simulink model "Quadrotor_SMC"  (R2021b)
settings: Solver=VariableStepAuto  StartTime=0.0  StopTime=10  RelTol=1e-3
undefined symbols (not defined in the file): e_Kp, K_rate_d, K_rate_p, Ki, Kp
libraries: simulink x2
settings Model: Creator=Biorobotic_MG  LastModifiedBy=Biorobotic_MG
settings DebuggingCC: UnderSpecifiedDimensionMsg=warning

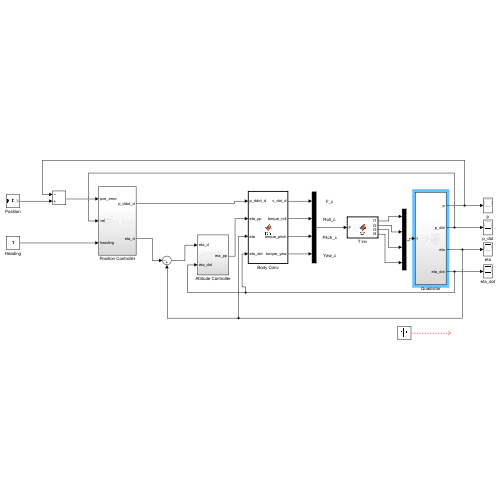
[thumbnail: Simulink's stored preview of the top-level diagram]
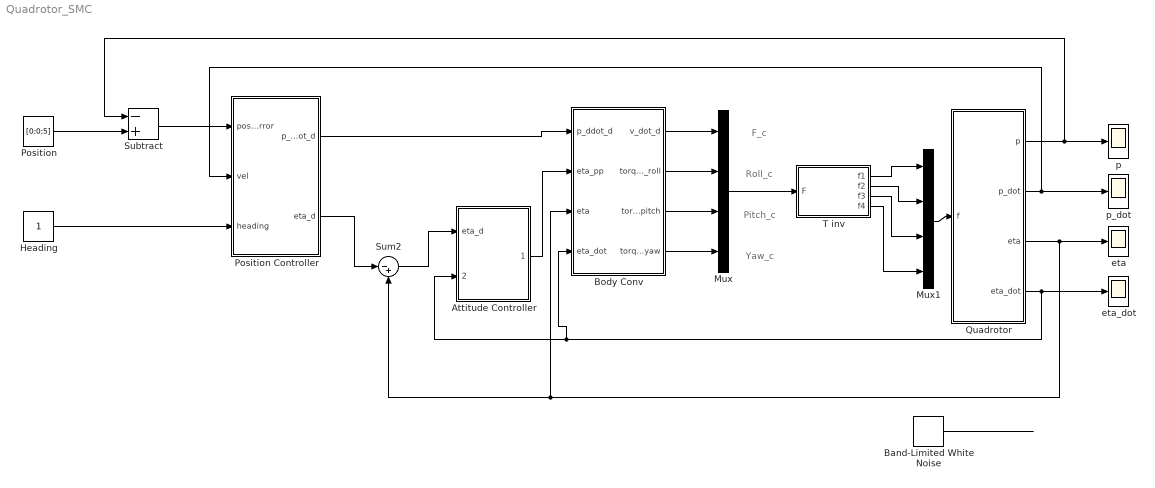
== system Quadrotor_SMC ==
  note: F_c
  note: Roll_c
  note: Pitch_c
  note: Yaw_c
  Attitude Controller : Subsystem
  Band-Limited White Noise : simulink/Sources/Band-Limited White Noise  Cov=[0.01]  Ts=0.1  seed=[23341]
  Body Conv : MATLAB Function  TreatAsAtomicUnit=on
  Heading : Constant
  Mux : Mux
  Mux1 : Mux
  Position : Constant  Value=[0;0;5]  VectorParams1D=off
  Position Controller : Subsystem
  Quadrotor : Subsystem
  Subtract : Sum  Inputs=-+
  Sum2 : Sum  Inputs=|-+
  T inv : MATLAB Function  TreatAsAtomicUnit=on
  eta : Scope
  eta_dot : Scope
  p : Scope
  p_dot : Scope
  wires:
  Quadrotor/1(p) -> Subtract/1, p/1
  Quadrotor/3(eta) -> Sum2/2, Body Conv/3(eta), eta/1
  T inv/1(f1) -> Mux1/1
  T inv/2(f2) -> Mux1/2
  T inv/3(f3) -> Mux1/3
  T inv/4(f4) -> Mux1/4
  Mux1/1 -> Quadrotor/1(f)
  Position/1 -> Subtract/2
  Attitude Controller/1(eta_pp) -> Body Conv/2(eta_pp)
  Subtract/1 -> Position Controller/1(pos_error)
  Heading/1 -> Position Controller/3(heading)
  Position Controller/2(eta_d) -> Sum2/1
  Mux/1 -> T inv/1(F)
  Position Controller/1(p_ddot_d) -> Body Conv/1(p_ddot_d)
  Quadrotor/4(eta_dot) -> eta_dot/1, Body Conv/4(eta_dot), Attitude Controller/2(eta_dot)
  Quadrotor/2(p_dot) -> Position Controller/2(vel), p_dot/1
  Body Conv/4(torque_yaw) -> Mux/4
  Body Conv/3(torque_pitch) -> Mux/3
  Body Conv/2(torque_roll) -> Mux/2
  Body Conv/1(v_dot_d) -> Mux/1
  Sum2/1 -> Attitude Controller/1(eta_d)
  Band-Limited White Noise/1 -> ?

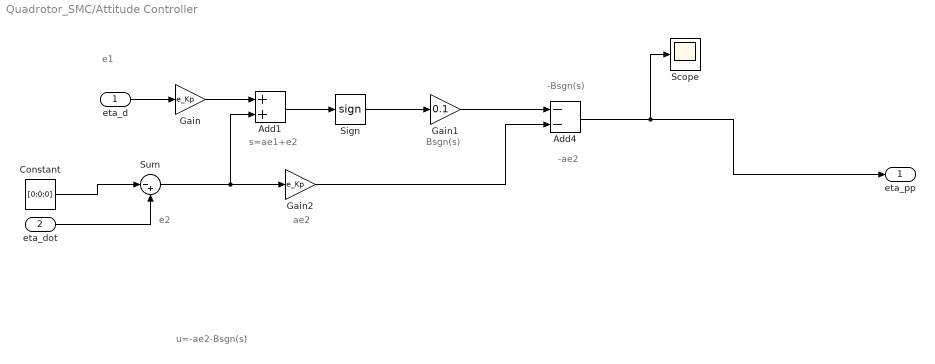
== system Quadrotor_SMC/Attitude Controller ==
  note: -ae2
  note: ae2
  note: e1
  note: e2
  note: s=ae1+e2
  note: Bsgn(s)
  note: -Bsgn(s)
  note: u=-ae2-Bsgn(s)
  eta_d : Inport
  eta_dot : Inport  Port=2
  Add1 : Sum
  Add4 : Sum  Inputs=--
  Constant : Constant  Value=[0;0;0]
  Gain : Gain  Gain=e_Kp
  Gain1 : Gain  Gain=0.1
  Gain2 : Gain  Gain=e_Kp
  Scope : Scope
  Sign : Signum  ZeroCross=off
  Sum : Sum  Inputs=|-+
  eta_pp : Outport
  wires:
  eta_d/1 -> Gain/1
  Gain/1 -> Add1/1
  Sign/1 -> Gain1/1
  Gain1/1 -> Add4/1
  Constant/1 -> Sum/1
  Add4/1 -> Scope/1, eta_pp/1
  Add1/1 -> Sign/1
  eta_dot/1 -> Sum/2
  Sum/1 -> Add1/2, Gain2/1
  Gain2/1 -> Add4/2

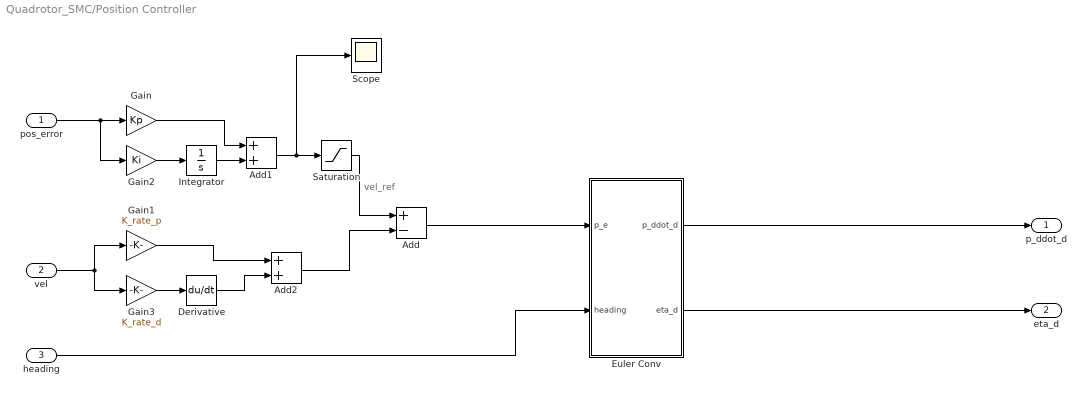
== system Quadrotor_SMC/Position Controller ==
  note: vel_ref
  pos_error : Inport
  vel : Inport  Port=2
  heading : Inport  Port=3
  Add : Sum  Inputs=+-
  Add1 : Sum
  Add2 : Sum
  Derivative : Derivative
  Euler Conv : MATLAB Function  TreatAsAtomicUnit=on
  Gain : Gain  Gain=Kp
  Gain1 : Gain  Gain=K_rate_p
  Gain2 : Gain  Gain=Ki
  Gain3 : Gain  Gain=K_rate_d
  Integrator : Integrator
  Saturation : Saturate  UpperLimit=3  LowerLimit=-3
  Scope : Scope
  p_ddot_d : Outport
  eta_d : Outport  Port=2
  wires:
  pos_error/1 -> Gain2/1, Gain/1
  Euler Conv/1(p_ddot_d) -> p_ddot_d/1
  heading/1 -> Euler Conv/2(heading)
  Gain/1 -> Add1/1
  Gain2/1 -> Integrator/1
  Integrator/1 -> Add1/2
  Gain3/1 -> Derivative/1
  vel/1 -> Gain1/1, Gain3/1
  Gain1/1 -> Add2/1
  Derivative/1 -> Add2/2
  Add2/1 -> Add/2
  Add/1 -> Euler Conv/1(p_e)
  Euler Conv/2(eta_d) -> eta_d/1
  Add1/1 -> Saturation/1, Scope/1
  Saturation/1 -> Add/1

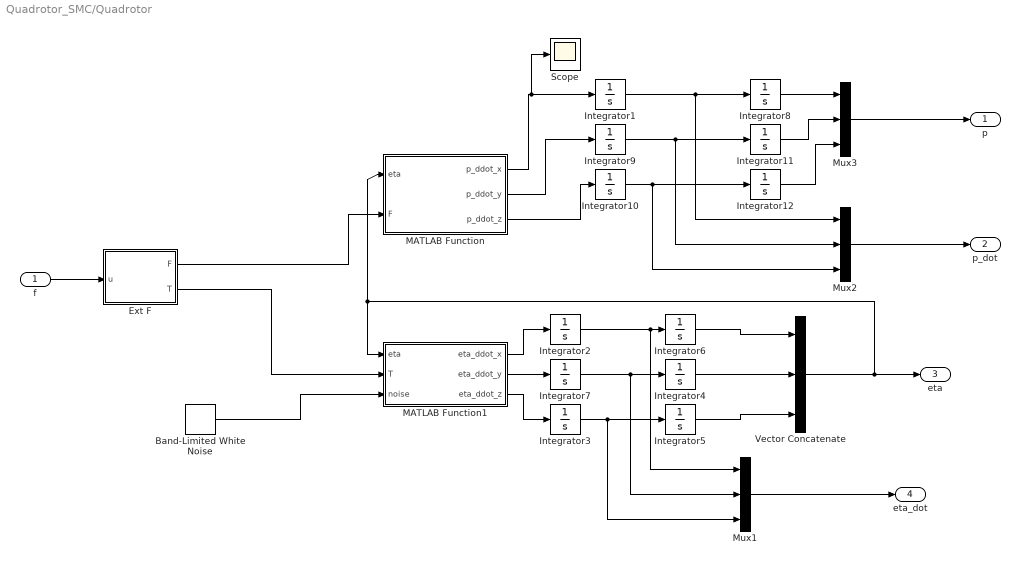
== system Quadrotor_SMC/Quadrotor ==
  f : Inport
  Band-Limited White Noise : simulink/Sources/Band-Limited White Noise  Cov=[0.01]  Ts=0.1  seed=[23341]
  Ext F : MATLAB Function  TreatAsAtomicUnit=on
  Integrator{1..12} (12 alike) : Integrator
  MATLAB Function : MATLAB Function  TreatAsAtomicUnit=on
  MATLAB Function1 : MATLAB Function  TreatAsAtomicUnit=on
  Mux1 : Mux  Inputs=3
  Mux2 : Mux  Inputs=3
  Mux3 : Mux  Inputs=3
  Scope : Scope
  Vector Concatenate : Concatenate  NumInputs=3  Mode=Multidimensional array
  p : Outport
  p_dot : Outport  Port=2
  eta : Outport  Port=3
  eta_dot : Outport  Port=4
  wires:
  Ext F/2(T) -> MATLAB Function1/2(T)
  Ext F/1(F) -> MATLAB Function/2(F)
  f/1 -> Ext F/1(u)
  Integrator10/1 -> Mux2/3, Integrator12/1
  Integrator12/1 -> Mux3/3
  Integrator11/1 -> Mux3/2
  Integrator9/1 -> Mux2/2, Integrator11/1
  Integrator1/1 -> Mux2/1, Integrator8/1
  MATLAB Function/1(p_ddot_x) -> Scope/1, Integrator1/1
  MATLAB Function/2(p_ddot_y) -> Integrator9/1
  MATLAB Function/3(p_ddot_z) -> Integrator10/1
  Integrator8/1 -> Mux3/1
  Mux3/1 -> p/1
  Mux2/1 -> p_dot/1
  Vector Concatenate/1 -> MATLAB Function/1(eta), MATLAB Function1/1(eta), eta/1
  MATLAB Function1/3(eta_ddot_z) -> Integrator3/1
  MATLAB Function1/2(eta_ddot_y) -> Integrator7/1
  Integrator4/1 -> Vector Concatenate/2
  Integrator6/1 -> Vector Concatenate/1
  Integrator2/1 -> Mux1/1, Integrator6/1
  Integrator7/1 -> Mux1/2, Integrator4/1
  Integrator3/1 -> Mux1/3, Integrator5/1
  Integrator5/1 -> Vector Concatenate/3
  MATLAB Function1/1(eta_ddot_x) -> Integrator2/1
  Mux1/1 -> eta_dot/1
  Band-Limited White Noise/1 -> MATLAB Function1/3(noise)

== matlab function Quadrotor_SMC/Quadrotor/MATLAB Function ==
  data: eta input; p_ddot_x output; F input; p_ddot_y output; p_ddot_z output
function [p_ddot_x, p_ddot_y, p_ddot_z] = fcn(eta, F)
m=1;
g=9.81;
%p_ddot = rand(3,1);
p_ddot_x=(1/m)*F*(sin(eta(1))*sin(eta(3)) + sin(eta(2))*cos(eta(1))*cos(eta(3)));
p_ddot_y=(1/m)*F*(-sin(eta(1))*cos(eta(3)) + sin(eta(3))*sin(eta(2))*cos(eta(1)));
p_ddot_z=(1/m)*(F)*cos(eta(1))*cos(eta(2))-g;

== matlab function Quadrotor_SMC/Quadrotor/Ext F ==
  data: u input; F output; T output
function [F,T] = fcn(u)
L=0.3;
g=9.81;
Fz= u(1)+u(2)+u(3)+u(4);
Tx= 0.707106781186547*L*(u(1)-u(2)-u(3)+u(4));
Ty= 0.707106781186547*L*(-u(1)-u(2)+u(3)+u(4));
Tz= 0.2*(+u(1)-u(2) +u(3) -u(4));
%Tz=0;

F = Fz;
T = [Tx;Ty;Tz];

== matlab function Quadrotor_SMC/Quadrotor/MATLAB Function1 ==
  data: eta input; T input; eta_ddot_x output; eta_ddot_y output; eta_ddot_z output; noise input
function [eta_ddot_x, eta_ddot_y, eta_ddot_z]  = fcn(eta,T,noise)
I_xx=0.04;
I_yy=0.04;
I_zz=0.006;
%eta_ddot = rand(3,1);

eta_ddot_x = (T(1) + T(3)*cos(eta(1))*tan(eta(2)) + T(2)*sin(eta(1))*tan(eta(2)))/I_xx + noise;
eta_ddot_y = (-T(3)*sin(eta(1)) + T(2)*cos(eta(1)))/I_yy + noise;
eta_ddot_z = (T(3)*cos(eta(1)) + T(2)*sin(eta(1)))/(I_zz*cos(eta(2))) + noise;

%eta_ddot = [eta_ddot_x;eta_ddot_y;eta_ddot_z];

== matlab function Quadrotor_SMC/T inv ==
  data: F input; f1 output; f2 output; f3 output; f4 output
function [f1,f2,f3,f4] = fcn(F)
L=0.3;
A=0.2;
f1=0.25*F(1) + 0.353553390593274*F(2)/L - 0.353553390593274*F(3)/L + 0.25*F(4)/A
f2=0.25*F(1) - 0.353553390593274*F(2)/L - 0.353553390593274*F(3)/L - 0.25*F(4)/A
f3=0.25*F(1) - 0.353553390593274*F(2)/L + 0.353553390593274*F(3)/L + 0.25*F(4)/A
f4=0.25*F(1) + 0.353553390593274*F(2)/L + 0.353553390593274*F(3)/L - 0.25*F(4)/A
%f = [0.25.*F(1) + 0.25.*d_p.*F(4)/b_p - 0.353553390593274.*F(2)/L + 0.353553390593274.*F(3)/L;
%    0.25.*F(1) - 0.25.*d_p.*F(4)/b_p + 0.353553390593274.*F(2)/L + 0.353553390593274.*F(3)/L;
%    0.25.*F(1) + 0.25.*d_p.*F(4)/b_p + 0.353553390593274.*F(2)/L - 0.353553390593274.*F(3)/L;
%    0.25.*F(1) - 0.25.*d_p.*F(4)/b_p - 0.353553390593274.*F(2)/L - 0.353553390593274.*F(3)/L];

== matlab function Quadrotor_SMC/Body Conv ==
  data: p_ddot_d input; v_dot_d output; eta_pp input; torque_roll output; eta input size=3; torque_pitch output; torque_yaw output; eta_dot input
function [v_dot_d,torque_roll, torque_pitch, torque_yaw]  = fcn(p_ddot_d,eta_pp,eta,eta_dot)
g=9.81;
I_xx=0.04;
I_yy=0.04;
I_zz=0.006;
v_dot_d=(p_ddot_d)*cos(eta(1))*cos(eta(2))%-g*cos(eta(1))*cos(eta(2));
%F = p*cos(eta(1))*cos(eta(2));
torque_roll = I_xx*eta_pp(1) - I_xx*eta_pp(3)*sin(eta(2));
torque_pitch = I_yy*eta_pp(3)*sin(eta(1))*cos(eta(2)) + I_yy*eta_pp(2)*cos(eta(1));
torque_yaw = I_zz*eta_pp(3)*cos(eta(1))*cos(eta(2)) - I_zz*eta_pp(2)*sin(eta(1));

%torque_roll = I_xx*(eta_dot(1)*eta_dot(2)*(I_yy - I_zz) + eta_pp(1) - (eta_dot(0)*eta_dot(1)*(I_yy - I_zz) + eta_pp(3))*sin(eta(2)));
%torque_pitch = I_yy*((eta_dot(0)*eta_dot(1)*(I_yy - I_zz) + eta_pp(3))*sin(eta(1))*cos(eta(2)) + (eta_dot(0)*eta_dot(2)*(I_yy - I_zz) + eta_pp(2))*cos(eta(1)));
%torque_yaw = I_zz*((eta_dot(0)*eta_dot(1)*(I_yy - I_zz) + eta_pp(3))*cos(eta(1))*cos(eta(2)) - (eta_dot(0)*eta_dot(2)*(I_yy - I_zz) + eta_pp(2))*sin(eta(1)));
%f = [0.25.*F(1) + 0.25.*d_p.*F(4)/b_p - 0.353553390593274.*F(2)/L + 0.353553390593274.*F(3)/L;
%    0.25.*F(1) - 0.25.*d_p.*F(4)/b_p + 0.353553390593274.*F(2)/L + 0.353553390593274.*F(3)/L;
%    0.25.*F(1) + 0.25.*d_p.*F(4)/b_p + 0.353553390593274.*F(2)/L - 0.353553390593274.*F(3)/L;
%    0.25.*F(1) - 0.25.*d_p.*F(4)/b_p - 0.353553390593274.*F(2)/L - 0.353553390593274.*F(3)/L];

== matlab function Quadrotor_SMC/Position Controller/Euler Conv ==
  data: p_e input; p_ddot_d output; eta_d output; heading input
function [p_ddot_d,eta_d] = fcn(p_e,heading)

g=9.81;
p_ddot_d =  p_e(3)+g;
phi_d = (p_e(1)*sin(heading)-p_e(2)*cos(heading)) /sqrt(p_e(1)^2+p_e(2)^2+(p_ddot_d)^2);
theta_d = (p_e(1)*cos(heading)+p_e(2)*sin(heading)) /(p_ddot_d);
%%%Navigation
%*cos(phi_d)*cos(theta_d);
%*cos(phi_d)*cos(theta_d)
eta_d = [phi_d; theta_d; heading];
